simulink library "EqMpro"  (R2021b)
settings: Solver=ode45  StartTime=0.0  StopTime=10.0  RelTol=1e-3  EnableMultiTasking=on
undefined symbols (not defined in the file or in its folder): g, p0, phi0, psi0, q0, r0, theta0, u0, v0, w0, X0, Y0, Z0
settings Model: Creator=bruno  LastModifiedBy=dmgp1
settings SolverCC: AlgebraicLoopSolver=TrustRegion
settings DataIOCC: LimitDataPoints=on  ReturnWorkspaceOutputs=off
settings OptimizationCC: LifeSpan=inf
settings DebuggingCC: AllowSymbolicDim=off  SFUnexpectedBacktrackingDiag=warning  SFNoUnconditionalDefaultTransitionDiag=warning  SFMachineParentedDataDiag=warning  ArithmeticOperatorsInVariantConditions=warning
settings SFSimCC: SimUseLocalCustomCode=off  CustomCodeUndefinedFunction=UseInterfaceOnly
settings RTWCC: RTWUseLocalCustomCode=off
settings CodeAppCC: StateflowObjectComments=on
settings GRTTargetCC: TargetLangStandard=C89/C90 (ANSI)
settings ConfigComp: CovMetricSettings=dw  CovSaveCumulativeToWorkspaceVar=on  CovSaveSingleToWorkspaceVar=on  CovExternalEMLEnable=off

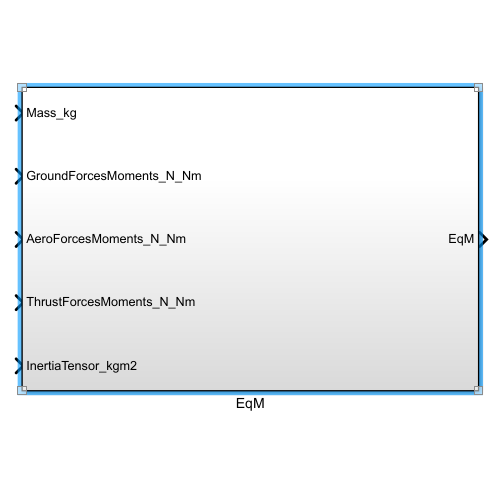
[thumbnail: Simulink's stored preview of the top-level diagram]
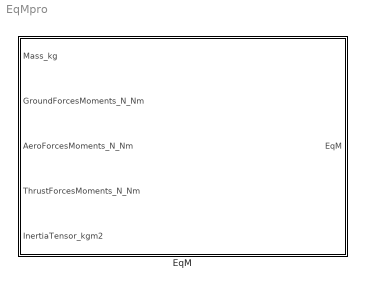
== system EqMpro ==
  EqM : Subsystem

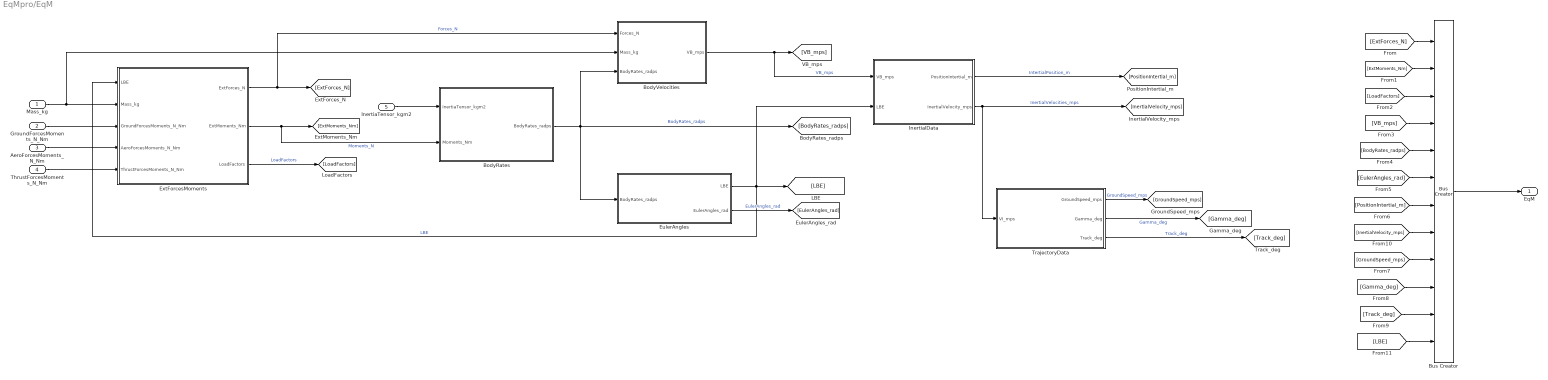
== system EqMpro/EqM ==
  Mass_kg : Inport
  GroundForcesMoments_N_Nm : Inport  Port=2
  AeroForcesMoments_N_Nm : Inport  Port=3
  ThrustForcesMoments_N_Nm : Inport  Port=4
  InertiaTensor_kgm2 : Inport  Port=5
  BodyRates : Subsystem
  BodyVelocities : Subsystem
  Bus Creator : BusCreator  Inputs=12
  EulerAngles : Subsystem
  ExtForcesMoments : Subsystem
  InertialData : Subsystem
  TrajectoryData : Subsystem
  EqM : Outport
  wires:
  [LBE] -> Bus Creator/12
  InertialData/1(PositionIntertial_m) -> [PositionIntertial_m]  "IntertialPosition_m"
  InertialData/2(InertialVelocity_mps) -> [InertialVelocity_mps], TrajectoryData/1(VI_mps)  "InertialVelocities_mps"
  [LoadFactors] -> Bus Creator/3
  [InertialVelocity_mps] -> Bus Creator/8
  ExtForcesMoments/2(ExtMoments_Nm) -> [ExtMoments_Nm], BodyRates/2(Moments_Nm)  "Moments_N"
  InertiaTensor_kgm2/1 -> BodyRates/1(InertiaTensor_kgm2)
  BodyRates/1(BodyRates_radps) -> [BodyRates_radps], EulerAngles/1(BodyRates_radps), BodyVelocities/3(BodyRates_radps)  "BodyRates_radps"
  ThrustForcesMoments_N_Nm/1 -> ExtForcesMoments/5(ThrustForcesMoments_N_Nm)
  GroundForcesMoments_N_Nm/1 -> ExtForcesMoments/3(GroundForcesMoments_N_Nm)
  EulerAngles/1(LBE) -> InertialData/2(LBE), ExtForcesMoments/1(LBE), [LBE]  "LBE"
  BodyVelocities/1(VB_mps) -> [VB_mps], InertialData/1(VB_mps)  "VB_mps"
  ExtForcesMoments/1(ExtForces_N) -> [ExtForces_N], BodyVelocities/1(Forces_N)  "Forces_N"
  Mass_kg/1 -> BodyVelocities/2(Mass_kg), ExtForcesMoments/2(Mass_kg)
  ExtForcesMoments/3(LoadFactors) -> [LoadFactors]  "LoadFactors"
  AeroForcesMoments_N_Nm/1 -> ExtForcesMoments/4(AeroForcesMoments_N_Nm)
  TrajectoryData/2(Gamma_deg) -> [Gamma_deg]  "Gamma_deg"
  TrajectoryData/3(Track_deg) -> [Track_deg]  "Track_deg"
  EulerAngles/2(EulerAngles_rad) -> [EulerAngles_rad]  "EulerAngles_rad"
  TrajectoryData/1(GroundSpeed_mps) -> [GroundSpeed_mps]  "GroundSpeed_mps"
  [GroundSpeed_mps] -> Bus Creator/9
  [Gamma_deg] -> Bus Creator/10
  [ExtMoments_Nm] -> Bus Creator/2
  [Track_deg] -> Bus Creator/11
  Bus Creator/1 -> EqM/1
  [ExtForces_N] -> Bus Creator/1
  [VB_mps] -> Bus Creator/4
  [BodyRates_radps] -> Bus Creator/5
  [EulerAngles_rad] -> Bus Creator/6
  [PositionIntertial_m] -> Bus Creator/7

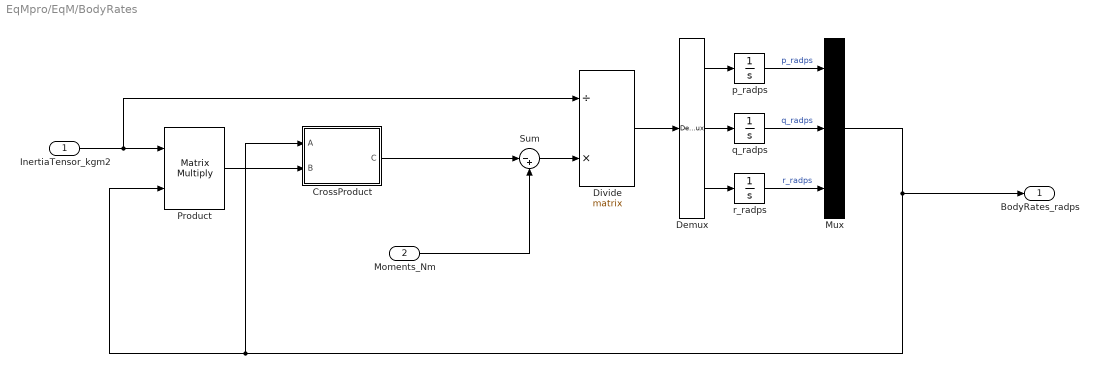
== system EqMpro/EqM/BodyRates ==
  InertiaTensor_kgm2 : Inport
  Moments_Nm : Inport  Port=2
  CrossProduct : Subsystem
  Demux : Demux  Outputs=3
  Divide : Product  Inputs=/*  Multiplication=Matrix(*)
  Mux : Mux  Inputs=3
  Product : Product  Multiplication=Matrix(*)
  Sum : Sum  Inputs=|-+
  p_radps : Integrator  InitialCondition=p0  ContinuousStateAttributes='p_radps'
  q_radps : Integrator  InitialCondition=q0  ContinuousStateAttributes='q_radps'
  r_radps : Integrator  InitialCondition=r0  ContinuousStateAttributes='r_radps'
  BodyRates_radps : Outport
  wires:
  r_radps/1 -> Mux/3  "r_radps"
  Mux/1 -> BodyRates_radps/1, CrossProduct/1(A), Product/2
  Sum/1 -> Divide/2
  p_radps/1 -> Mux/1  "p_radps"
  Product/1 -> CrossProduct/2(B)
  Moments_Nm/1 -> Sum/2
  CrossProduct/1(C) -> Sum/1
  q_radps/1 -> Mux/2  "q_radps"
  InertiaTensor_kgm2/1 -> Divide/1, Product/1
  Demux/1 -> p_radps/1
  Demux/3 -> r_radps/1
  Demux/2 -> q_radps/1
  Divide/1 -> Demux/1

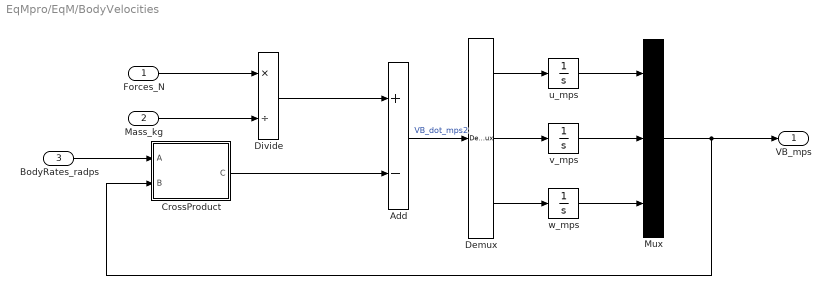
== system EqMpro/EqM/BodyVelocities ==
  Forces_N : Inport
  Mass_kg : Inport  Port=2
  BodyRates_radps : Inport  Port=3
  Add : Sum  Inputs=+-
  CrossProduct : Subsystem
  Demux : Demux  Outputs=3
  Divide : Product  Inputs=*/
  Mux : Mux  Inputs=3
  u_mps : Integrator  InitialCondition=u0  ContinuousStateAttributes='u_mps'
  v_mps : Integrator  InitialCondition=v0  ContinuousStateAttributes='v_mps'
  w_mps : Integrator  InitialCondition=w0  ContinuousStateAttributes='w_mps'
  VB_mps : Outport
  wires:
  Divide/1 -> Add/1
  Add/1 -> Demux/1  "VB_dot_mps2"
  Forces_N/1 -> Divide/1
  Mux/1 -> CrossProduct/2(B), VB_mps/1
  BodyRates_radps/1 -> CrossProduct/1(A)
  CrossProduct/1(C) -> Add/2
  Demux/1 -> u_mps/1
  v_mps/1 -> Mux/2
  w_mps/1 -> Mux/3
  Demux/2 -> v_mps/1
  Demux/3 -> w_mps/1
  u_mps/1 -> Mux/1
  Mass_kg/1 -> Divide/2

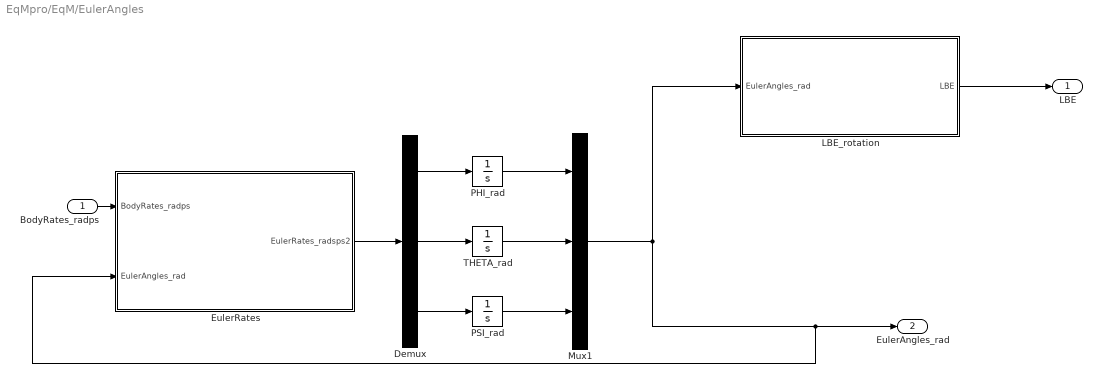
== system EqMpro/EqM/EulerAngles ==
  BodyRates_radps : Inport
  Demux : Demux  Outputs=3
  EulerRates : Subsystem
  LBE_rotation : Subsystem
  Mux1 : Mux  Inputs=3
  PHI_rad : Integrator  InitialCondition=phi0  ContinuousStateAttributes='PHI_rad'
  PSI_rad : Integrator  InitialCondition=psi0  ContinuousStateAttributes='PSI_rad'
  THETA_rad : Integrator  InitialCondition=theta0  ContinuousStateAttributes='THETA_rad'
  LBE : Outport
  EulerAngles_rad : Outport  Port=2
  wires:
  Demux/2 -> THETA_rad/1
  Demux/3 -> PSI_rad/1
  PHI_rad/1 -> Mux1/1
  THETA_rad/1 -> Mux1/2
  PSI_rad/1 -> Mux1/3
  Mux1/1 -> EulerRates/2(EulerAngles_rad), EulerAngles_rad/1, LBE_rotation/1(EulerAngles_rad)
  Demux/1 -> PHI_rad/1
  EulerRates/1(EulerRates_radsps2) -> Demux/1
  LBE_rotation/1(LBE) -> LBE/1
  BodyRates_radps/1 -> EulerRates/1(BodyRates_radps)

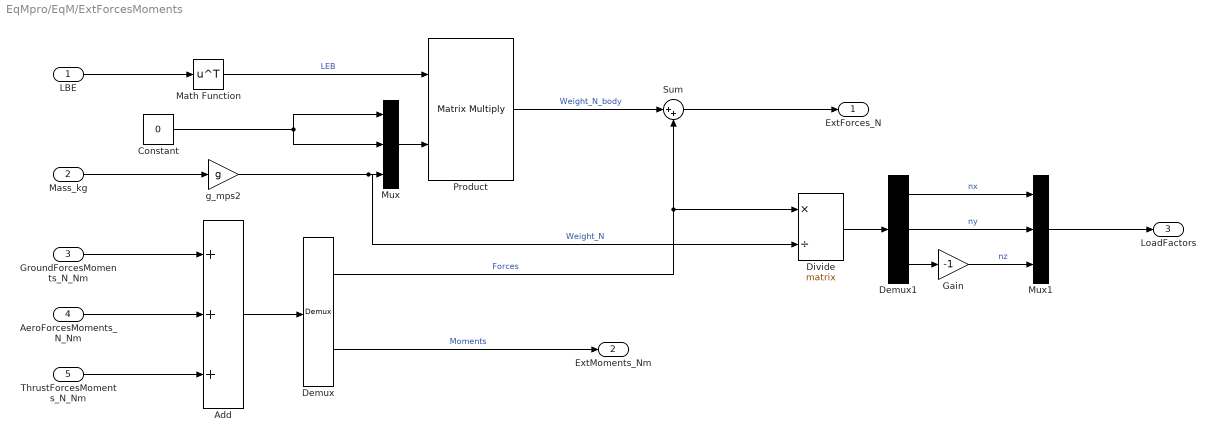
== system EqMpro/EqM/ExtForcesMoments ==
  LBE : Inport
  Mass_kg : Inport  Port=2
  GroundForcesMoments_N_Nm : Inport  Port=3
  AeroForcesMoments_N_Nm : Inport  Port=4
  ThrustForcesMoments_N_Nm : Inport  Port=5
  Add : Sum  Inputs=+++
  Constant : Constant  Value=0
  Demux : Demux  Outputs=2
  Demux1 : Demux  Outputs=3
  Divide : Product  Inputs=*/  Multiplication=Matrix(*)
  Gain : Gain  Gain=-1
  Math Function : Math  Operator=transpose  SignedPower=on  SaturateOnIntegerOverflow=on
  Mux : Mux  Inputs=3
  Mux1 : Mux  Inputs=3
  Product : Product  Multiplication=Matrix(*)
  Sum : Sum  Inputs=|++
  g_mps2 : Gain  Gain=g
  ExtForces_N : Outport
  ExtMoments_Nm : Outport  Port=2
  LoadFactors : Outport  Port=3
  wires:
  Demux/1 -> Sum/2, Divide/1  "Forces"
  Math Function/1 -> Product/1  "LEB"
  GroundForcesMoments_N_Nm/1 -> Add/1
  Constant/1 -> Mux/2, Mux/1
  Demux/2 -> ExtMoments_Nm/1  "Moments"
  Gain/1 -> Mux1/3  "nz"
  Demux1/3 -> Gain/1
  Mux1/1 -> LoadFactors/1
  AeroForcesMoments_N_Nm/1 -> Add/2
  Demux1/2 -> Mux1/2  "ny"
  Demux1/1 -> Mux1/1  "nx"
  Mass_kg/1 -> g_mps2/1
  g_mps2/1 -> Divide/2, Mux/3  "Weight_N"
  LBE/1 -> Math Function/1
  Add/1 -> Demux/1
  Mux/1 -> Product/2
  ThrustForcesMoments_N_Nm/1 -> Add/3
  Divide/1 -> Demux1/1
  Sum/1 -> ExtForces_N/1
  Product/1 -> Sum/1  "Weight_N_body"

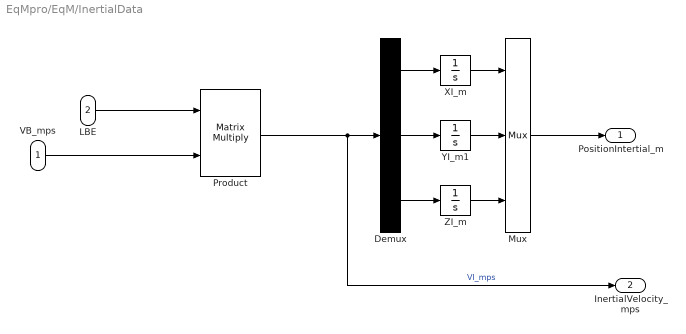
== system EqMpro/EqM/InertialData ==
  VB_mps : Inport
  LBE : Inport  Port=2
  Demux : Demux  Outputs=3
  Mux : Mux  Inputs=3
  Product : Product  Multiplication=Matrix(*)
  XI_m : Integrator  InitialCondition=X0  ContinuousStateAttributes='XI_m'
  YI_m1 : Integrator  InitialCondition=Y0  ContinuousStateAttributes='YI_m'
  ZI_m : Integrator  InitialCondition=Z0  ContinuousStateAttributes='ZI_m'
  PositionIntertial_m : Outport
  InertialVelocity_mps : Outport  Port=2
  wires:
  LBE/1 -> Product/1
  VB_mps/1 -> Product/2
  Mux/1 -> PositionIntertial_m/1
  YI_m1/1 -> Mux/2
  XI_m/1 -> Mux/1
  ZI_m/1 -> Mux/3
  Product/1 -> InertialVelocity_mps/1, Demux/1  "VI_mps"
  Demux/1 -> XI_m/1
  Demux/2 -> YI_m1/1
  Demux/3 -> ZI_m/1

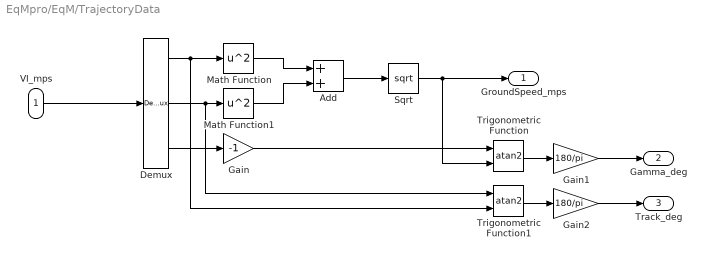
== system EqMpro/EqM/TrajectoryData ==
  VI_mps : Inport
  Add : Sum
  Demux : Demux  Outputs=3
  Gain : Gain  Gain=-1
  Gain1 : Gain  Gain=180/pi
  Gain2 : Gain  Gain=180/pi
  Math Function : Math  Operator=square  SignedPower=on  SaturateOnIntegerOverflow=on
  Math Function1 : Math  Operator=square  SignedPower=on  SaturateOnIntegerOverflow=on
  Sqrt : Sqrt  SaturateOnIntegerOverflow=on
  Trigonometric Function : Trigonometry  Operator=atan2
  Trigonometric Function1 : Trigonometry  Operator=atan2
  GroundSpeed_mps : Outport
  Gamma_deg : Outport  Port=2
  Track_deg : Outport  Port=3
  wires:
  Gain2/1 -> Track_deg/1
  Gain1/1 -> Gamma_deg/1
  Math Function/1 -> Add/1
  Math Function1/1 -> Add/2
  Trigonometric Function/1 -> Gain1/1
  Demux/3 -> Gain/1
  Demux/2 -> Trigonometric Function1/1, Math Function1/1
  Sqrt/1 -> GroundSpeed_mps/1, Trigonometric Function/2
  Demux/1 -> Trigonometric Function1/2, Math Function/1
  Add/1 -> Sqrt/1
  Gain/1 -> Trigonometric Function/1
  Trigonometric Function1/1 -> Gain2/1
  VI_mps/1 -> Demux/1

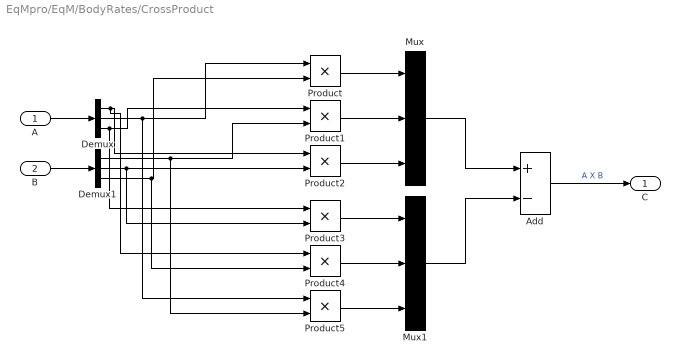
== system EqMpro/EqM/BodyRates/CrossProduct ==
  A : Inport
  B : Inport  Port=2
  Add : Sum  Inputs=+-
  Demux : Demux  Outputs=3
  Demux1 : Demux  Outputs=3
  Mux : Mux  Inputs=3
  Mux1 : Mux  Inputs=3
  Product{,1..5} (6 alike) : Product
  C : Outport
  wires:
  Product4/1 -> Mux1/2
  Demux1/3 -> Product4/2, Product/2
  Product1/1 -> Mux/2
  Product5/1 -> Mux1/3
  Mux/1 -> Add/1
  Demux1/1 -> Product5/2, Product1/2
  Product3/1 -> Mux1/1
  A/1 -> Demux/1
  Demux/2 -> Product5/1, Product/1
  Mux1/1 -> Add/2
  B/1 -> Demux1/1
  Demux/3 -> Product3/1, Product1/1
  Demux1/2 -> Product3/2, Product2/2
  Demux/1 -> Product4/1, Product2/1
  Product/1 -> Mux/1
  Product2/1 -> Mux/3
  Add/1 -> C/1  "A X B"

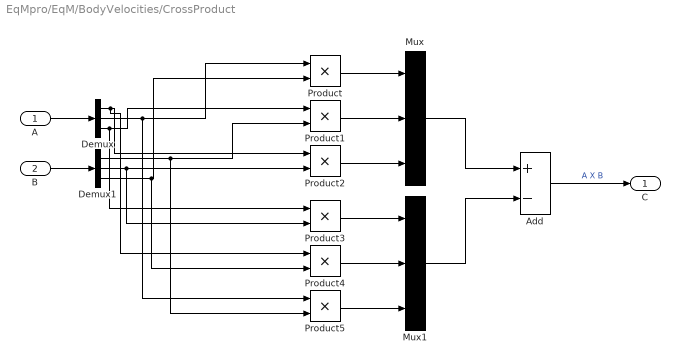
== system EqMpro/EqM/BodyVelocities/CrossProduct ==
  A : Inport
  B : Inport  Port=2
  Add : Sum  Inputs=+-
  Demux : Demux  Outputs=3
  Demux1 : Demux  Outputs=3
  Mux : Mux  Inputs=3
  Mux1 : Mux  Inputs=3
  Product{,1..5} (6 alike) : Product
  C : Outport
  wires:
  Product4/1 -> Mux1/2
  Demux1/3 -> Product4/2, Product/2
  Product1/1 -> Mux/2
  Product5/1 -> Mux1/3
  Mux/1 -> Add/1
  Demux1/1 -> Product5/2, Product1/2
  Product3/1 -> Mux1/1
  A/1 -> Demux/1
  Demux/2 -> Product5/1, Product/1
  Mux1/1 -> Add/2
  B/1 -> Demux1/1
  Demux/3 -> Product3/1, Product1/1
  Demux1/2 -> Product3/2, Product2/2
  Demux/1 -> Product4/1, Product2/1
  Product/1 -> Mux/1
  Product2/1 -> Mux/3
  Add/1 -> C/1  "A X B"

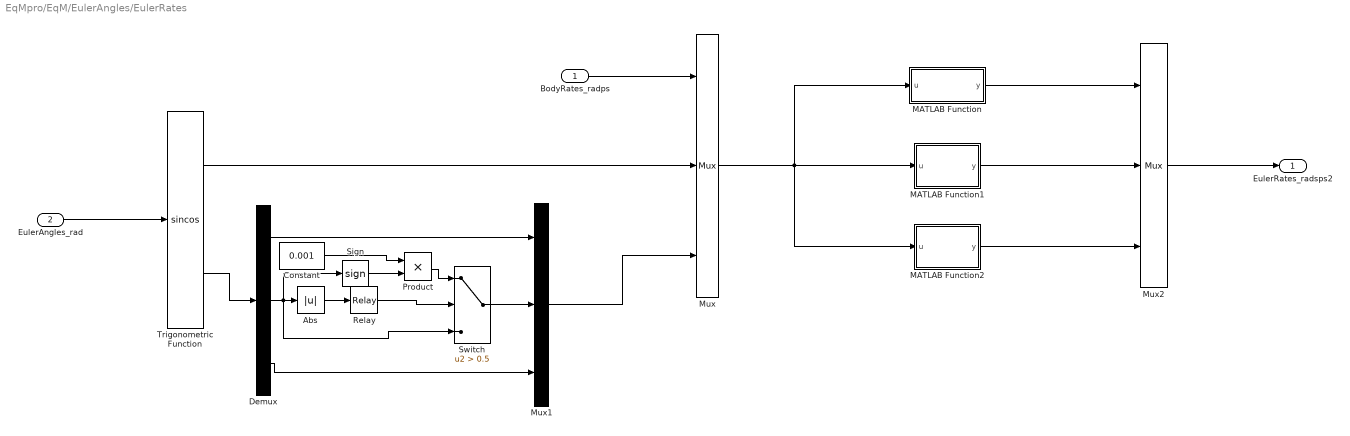
== system EqMpro/EqM/EulerAngles/EulerRates ==
  BodyRates_radps : Inport
  EulerAngles_rad : Inport  Port=2
  Abs : Abs
  Constant : Constant  Value=0.001
  Demux : Demux  Outputs=3
  MATLAB Function : MATLAB Function  TreatAsAtomicUnit=on
  MATLAB Function1 : MATLAB Function  TreatAsAtomicUnit=on
  MATLAB Function2 : MATLAB Function  TreatAsAtomicUnit=on
  Mux : Mux  Inputs=3
  Mux1 : Mux  Inputs=3
  Mux2 : Mux  Inputs=3
  Product : Product
  Relay : Relay  OnSwitchValue=.001  OffSwitchValue=0  OnOutputValue=0  OffOutputValue=1
  Sign : Signum
  Switch : Switch  Criteria=u2 > Threshold  Threshold=0.5
  Trigonometric Function : Trigonometry  Operator=sincos
  EulerRates_radsps2 : Outport
  wires:
  Mux/1 -> MATLAB Function/1(u), MATLAB Function1/1(u), MATLAB Function2/1(u)
  EulerAngles_rad/1 -> Trigonometric Function/1
  Trigonometric Function/2 -> Demux/1
  Demux/1 -> Mux1/1
  Relay/1 -> Switch/2
  BodyRates_radps/1 -> Mux/1
  MATLAB Function/1(y) -> Mux2/1
  MATLAB Function1/1(y) -> Mux2/2
  Abs/1 -> Relay/1
  Product/1 -> Switch/1
  MATLAB Function2/1(y) -> Mux2/3
  Mux2/1 -> EulerRates_radsps2/1
  Demux/2 -> Sign/1, Abs/1, Switch/3
  Switch/1 -> Mux1/2
  Sign/1 -> Product/2
  Constant/1 -> Product/1
  Demux/3 -> Mux1/3
  Trigonometric Function/1 -> Mux/2
  Mux1/1 -> Mux/3

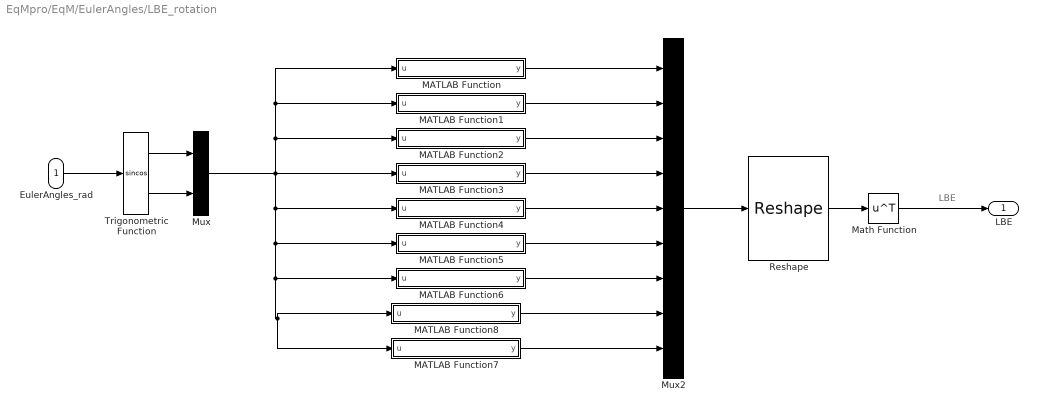
== system EqMpro/EqM/EulerAngles/LBE_rotation ==
  note: LBE
  EulerAngles_rad : Inport
  MATLAB Function : MATLAB Function  TreatAsAtomicUnit=on
  MATLAB Function1 : MATLAB Function  TreatAsAtomicUnit=on
  MATLAB Function2 : MATLAB Function  TreatAsAtomicUnit=on
  MATLAB Function3 : MATLAB Function  TreatAsAtomicUnit=on
  MATLAB Function4 : MATLAB Function  TreatAsAtomicUnit=on
  MATLAB Function5 : MATLAB Function  TreatAsAtomicUnit=on
  MATLAB Function6 : MATLAB Function  TreatAsAtomicUnit=on
  MATLAB Function7 : MATLAB Function  TreatAsAtomicUnit=on
  MATLAB Function8 : MATLAB Function  TreatAsAtomicUnit=on
  Math Function : Math  Operator=transpose  SignedPower=on  SaturateOnIntegerOverflow=on
  Mux : Mux  Inputs=2
  Mux2 : Mux  Inputs=9
  Reshape : Reshape  OutputDimensionality=Customize  OutputDimensions=[3,3]
  Trigonometric Function : Trigonometry  Operator=sincos
  LBE : Outport
  wires:
  MATLAB Function4/1(y) -> Mux2/5
  EulerAngles_rad/1 -> Trigonometric Function/1
  Trigonometric Function/2 -> Mux/2
  Mux2/1 -> Reshape/1
  Reshape/1 -> Math Function/1
  Math Function/1 -> LBE/1
  MATLAB Function2/1(y) -> Mux2/3
  MATLAB Function3/1(y) -> Mux2/4
  MATLAB Function/1(y) -> Mux2/1
  MATLAB Function1/1(y) -> Mux2/2
  Trigonometric Function/1 -> Mux/1
  Mux/1 -> MATLAB Function/1(u), MATLAB Function1/1(u), MATLAB Function2/1(u), MATLAB Function8/1(u), MATLAB Function7/1(u), MATLAB Function6/1(u), MATLAB Function5/1(u), MATLAB Function4/1(u), MATLAB Function3/1(u)
  MATLAB Function5/1(y) -> Mux2/6
  MATLAB Function6/1(y) -> Mux2/7
  MATLAB Function8/1(y) -> Mux2/8
  MATLAB Function7/1(y) -> Mux2/9

== matlab function EqMpro/EqM/EulerAngles/EulerRates/MATLAB Function ==
  data: u input size=[9]; y output size=[1]
function y = fcn(u)

y = u(1)+u(2)*u(4)*(u(5)/u(8))+u(3)*u(7)*(u(5)/u(8));

== matlab function EqMpro/EqM/EulerAngles/EulerRates/MATLAB Function2 ==
  data: u input size=[9]; y output size=[1]
function y = fcn(u)

y = (u(2)*u(4)+u(3)*u(7))/u(8);

== matlab function EqMpro/EqM/EulerAngles/LBE_rotation/MATLAB Function ==
  data: u input size=[6]; y output size=[1]
function y = fcn(u)

y = u(5)*u(6);

== matlab function EqMpro/EqM/EulerAngles/LBE_rotation/MATLAB Function1 ==
  data: u input size=[6]; y output size=[1]
function y = fcn(u)

y = u(1)*u(2)*u(6) - u(4)*u(3);

== matlab function EqMpro/EqM/EulerAngles/LBE_rotation/MATLAB Function2 ==
  data: u input size=[6]; y output size=[1]
function y = fcn(u)

y = u(6)*u(2)*u(4) + u(1)*u(3);

== matlab function EqMpro/EqM/EulerAngles/LBE_rotation/MATLAB Function3 ==
  data: u input size=[6]; y output size=[1]
function y = fcn(u)

y = u(5)*u(3);

== matlab function EqMpro/EqM/EulerAngles/LBE_rotation/MATLAB Function4 ==
  data: u input size=[6]; y output size=[1]
function y = fcn(u)

y = u(1)*u(2)*u(3) + u(4)*u(6);

== matlab function EqMpro/EqM/EulerAngles/LBE_rotation/MATLAB Function5 ==
  data: u input size=[6]; y output size=[1]
function y = fcn(u)

y = u(4)*u(2)*u(3) -u(1)*u(6);

== matlab function EqMpro/EqM/EulerAngles/EulerRates/MATLAB Function1 ==
  data: u input size=[9]; y output size=[1]
function y = fcn(u)

y = u(2)*u(7)-u(3)*u(4);

== matlab function EqMpro/EqM/EulerAngles/LBE_rotation/MATLAB Function6 ==
  data: u input size=[6]; y output size=[1]
function y = fcn(u)

y = -u(2);

== matlab function EqMpro/EqM/EulerAngles/LBE_rotation/MATLAB Function7 ==
  data: u input size=[6]; y output size=[1]
function y = fcn(u)

y = u(4)*u(5);

== matlab function EqMpro/EqM/EulerAngles/LBE_rotation/MATLAB Function8 ==
  data: u input size=[6]; y output size=[1]
function y = fcn(u)

y = u(1)*u(5);
